simulink model "washingMAchine"  (R2023b)
settings: Solver=FixedStepDiscrete  StartTime=0.0  StopTime=1.5  FixedStep=0.01  RelTol=1e-3
settings Model: Creator=Pranav  LastModifiedBy=Pranav

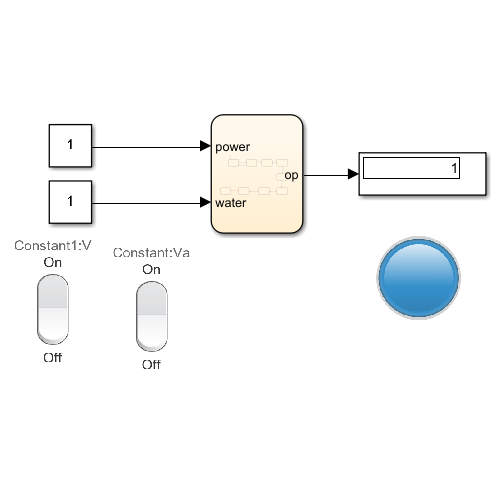
[thumbnail: Simulink's stored preview of the top-level diagram]
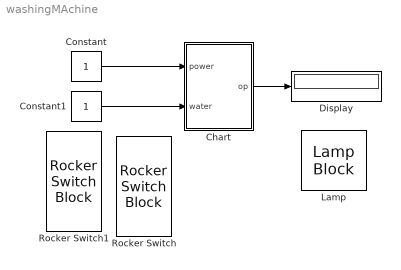
== system washingMAchine ==
  Chart : Stateflow chart  TreatAsAtomicUnit=on
  Constant : Constant
  Constant1 : Constant
  Display : Display
  Lamp : LampBlock  LabelPosition=Hide
  Rocker Switch : RockerSwitchBlock
      settings: Values={{'Off', 'On'}, [0 1]}
  Rocker Switch1 : RockerSwitchBlock
      settings: Values={{'Off', 'On'}, [0 1]}
  wires:
  Constant/1 -> Chart/1(power)
  Constant1/1 -> Chart/2(water)
  Chart/1(op) -> Display/1

== stateflow chart washingMAchine/Chart ==
  state off
    op=0;
  state idle
    op=1;
  state fillWater
    op=2;
  state heatingWater
    op=3;
  state washing
    op=4;
  state Finish
    op=8;
  state Spinning
    op=7;
  state Rinse
    op=6;
  state HeatingforRinse
    op=5;
  (default) -> off
  idle -> fillWater [order 2] : [water==1]
  fillWater -> heatingWater : after(0.1,sec)
  off -> idle : [power ==1]
  idle -> off [order 1] : [power ==0]
  heatingWater -> washing : after(0.25,sec)
  washing -> HeatingforRinse : after(0.25,sec)
  Spinning -> ? : after(0.3,sec)
  Rinse -> Spinning : after(0.2,sec)
  HeatingforRinse -> Rinse : after(0.3,sec)
  data: power input; water input; op output
